simulink model "identifikaciaa"  (R2021a)
settings: Solver=FixedStepAuto  StartTime=0.0  StopTime=stopTime  FixedStep=Ts  RelTol=1e-3
values from neighbouring files (symbols this model uses):
  den = [a2, a1, a0]    [identFitS.m]    (also in srdce.m; tlak.m = [a3, a2, a1, a0])
  initVal = 5.6    [srdce.m]    (also in tlak.m = pFilter(tLvzorka))
  num = [b1, b0]    [identFitS.m]    (also in srdce.m; tlak.m = [b2, b1, b0])
  stepTime = 150    [srdce.m]    (also in tlak.m = 133)
settings Model: Creator=marko  LastModifiedBy=marko

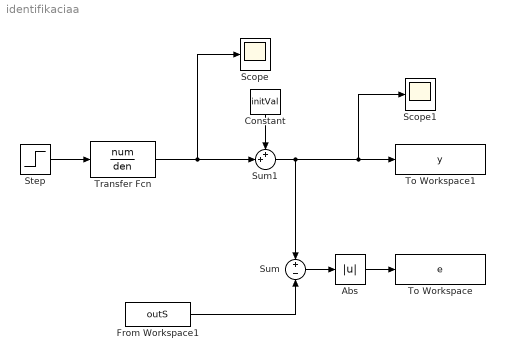
== system identifikaciaa ==
  Abs : Abs
  Constant : Constant  Value=initVal
  From Workspace1 : FromWorkspace  VariableName=outS  Interpolate=off  OutputAfterFinalValue=Holding final value
  Scope : Scope
  Scope1 : Scope
  Step : Step  Time=stepTime  After=-1  SampleTime=0
  Sum : Sum  Inputs=+|-
  Sum1 : Sum  Inputs=++|
  To Workspace : ToWorkspace  VariableName=e  SampleTime=-1
  To Workspace1 : ToWorkspace  VariableName=y  SaveFormat=Timeseries  SampleTime=-1
  Transfer Fcn : TransferFcn  Numerator=num  Denominator=den
  wires:
  From Workspace1/1 -> Sum/2
  Sum/1 -> Abs/1
  Abs/1 -> To Workspace/1
  Step/1 -> Transfer Fcn/1
  Transfer Fcn/1 -> Scope/1, Sum1/2
  Sum1/1 -> Sum/1, Scope1/1, To Workspace1/1
  Constant/1 -> Sum1/1
